simulink model "NL_MSD_RefTrajTrac_Opti_FeedBack_Lin_v01"  (R2024b)
settings: Solver=VariableStepAuto  StartTime=0.0  StopTime=Tend  RelTol=1e-3
values from neighbouring files (symbols this model uses):
  c = zeta * ccr    [Trajectory_Profile_v01.m]
  k = 1e3    (= 1000)    [Trajectory_Profile_v01.m]
  m = 1    [Trajectory_Profile_v01.m]
undefined symbols (not defined in the file or in its folder): aa1, aa2, aa3
settings Model: Creator=ababaei  LastModifiedBy=ababaei

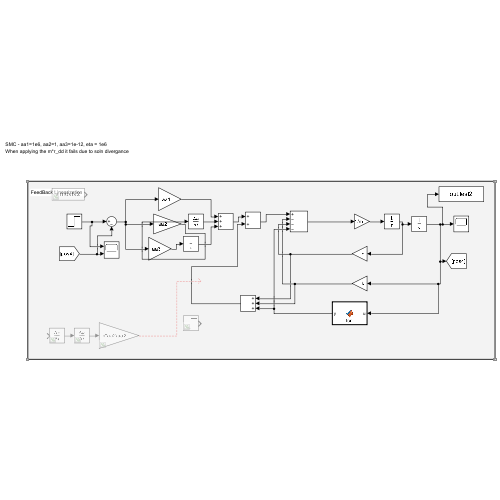
[thumbnail: Simulink's stored preview of the top-level diagram]
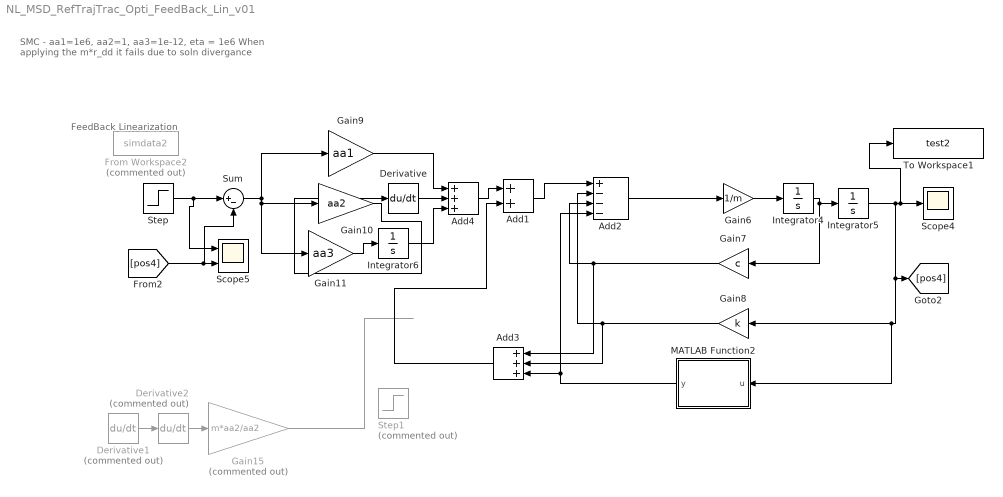
== system NL_MSD_RefTrajTrac_Opti_FeedBack_Lin_v01 ==
  note: FeedBack Linearization
  note: SMC - aa1=1e6, aa2=1, aa3=1e-12, eta = 1e6
      | When applying the m*r_dd it fails due to soln divergance
  Add1 : Sum
  Add2 : Sum  Inputs=+---
  Add3 : Sum  Inputs=+++
  Add4 : Sum  Inputs=+++
  Derivative : Derivative
  Derivative1 : Derivative  Commented=on
  Derivative2 : Derivative  Commented=on
  From Workspace2 : FromWorkspace  Commented=on  VariableName=simdata2
  Gain10 : Gain  Gain=aa2
  Gain11 : Gain  Gain=aa3
  Gain15 : Gain  Commented=on  Gain=m*aa2/aa2
  Gain6 : Gain  Gain=1/m
  Gain7 : Gain  Gain=c
  Gain8 : Gain  Gain=k
  Gain9 : Gain  Gain=aa1
  Integrator4 : Integrator
  Integrator5 : Integrator
  Integrator6 : Integrator
  MATLAB Function2 : MATLAB Function  TreatAsAtomicUnit=on
  Scope4 : Scope
  Scope5 : Scope  NumInputPorts=2
  Step : Step  Time=0.2  SampleTime=0
  Step1 : Step  Commented=on  Time=0.1  SampleTime=0
  Sum : Sum  Inputs=|+-
  To Workspace1 : ToWorkspace  VariableName=test2  SaveFormat=Timeseries  SampleTime=-1
  wires:
  Gain11/1 -> Integrator6/1
  Gain15/1 -> ?
  Integrator4/1 -> Integrator5/1, Gain7/1
  Derivative/1 -> Add4/2
  Add2/1 -> Gain6/1
  Step/1 -> Scope5/1, Sum/1
  Derivative1/1 -> Derivative2/1
  Sum/1 -> Gain11/1, Gain10/1, Gain9/1
  Add3/1 -> Add1/2
  Integrator6/1 -> Add4/3
  Gain6/1 -> Integrator4/1
  Derivative2/1 -> Gain15/1
  Gain9/1 -> Add4/1
  Gain10/1 -> Derivative/1
  Add4/1 -> Add1/1
  Add1/1 -> Add2/1
  [pos4] -> Sum/2, Scope5/2
  Integrator5/1 -> MATLAB Function2/1(u), Gain8/1, [pos4], To Workspace1/1, Scope4/1
  MATLAB Function2/1(y) -> Add3/3, Add2/4
  Gain8/1 -> Add3/2, Add2/2
  Gain7/1 -> Add3/1, Add2/3

== matlab function NL_MSD_RefTrajTrac_Opti_FeedBack_Lin_v01/MATLAB Function2 ==
  data: u input; y output
function y = fcn(u)
kNL = 100;
y = kNL*u;
